simulink library "sm_cable_robot_lib"  (R2021b)
settings: Solver=VariableStepAuto  StartTime=0.0  StopTime=10.0  RelTol=1e-3
undefined symbols (not defined in the file or in its folder): Hand, Left, Right, X, Y, Z
libraries: sm_lib x71, $bdroot x22
(part 1 of 3)
Description:
  | Cable Robot Library
settings Model: Creator=The MathWorks, Inc.  LastModifiedBy=The MathWorks, Inc.
settings SolverCC: AlgebraicLoopSolver=TrustRegion  DecoupledContinuousIntegration=on  MinimalZcImpactIntegration=on
settings DataIOCC: ReturnWorkspaceOutputs=off
settings DebuggingCC: SFMachineParentedDataDiag=warning  ArithmeticOperatorsInVariantConditions=warning
settings SFSimCC: SimUseLocalCustomCode=off  CustomCodeUndefinedFunction=UseInterfaceOnly
settings RTWCC: RTWUseLocalCustomCode=off

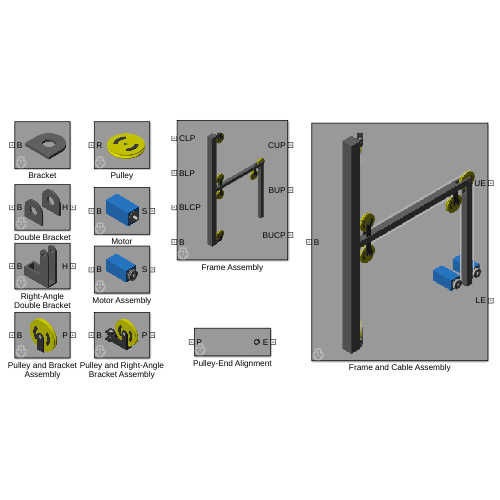
[thumbnail: Simulink's stored preview of the top-level diagram]
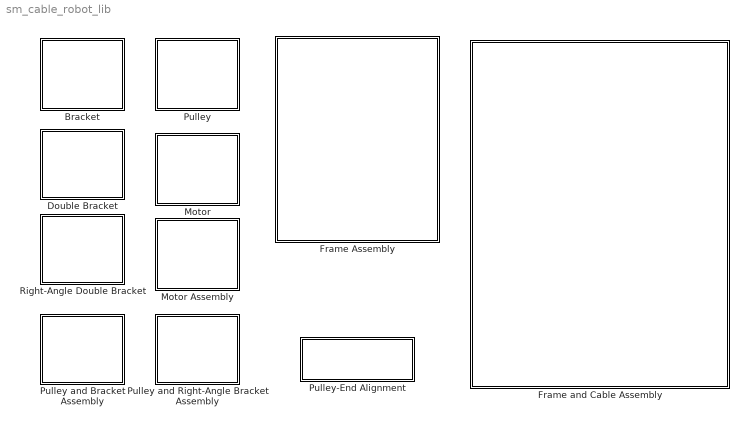
== system sm_cable_robot_lib ==
  Bracket : Subsystem  mask(Bracket){height=0.1, width=0.1, thickness=0.01, holeOffset=0.05, holeRadius=0.02, rho=2700, color=[0.5 0.5 0.5]}
      mask prompts: height "Height (m)"; width "Width (m)"; thickness "Thickness (m)"; holeOffset "Hole Offset (m)"; holeRadius "Hole Radius (m)"; rho "Density (kg/m^3)"; color "Color [r g b]"
      mask help:
      | This block models a bracket element.
      |
      | Port B corresponds to the center point of the base face.
      mask init:
      | y = height - 0.5*width;
      | 
      | outerVertices = ...
      |   [          0      0;...
      |      0.5*width      0;...
      |      0.5*width      y;...
      |      0.5*width height;...
      |     -0.5*width height;...
      |     -0.5*width      y;...
      |     -0.5*width      0;...
      |              0      0];
      | 
      | outer = simmechanics.demohelpers.round_corners(...
      |   outerVertices, [4 5], 0.5*width, 10);
      | 
      | holeTheta = linspace(1.5*pi, -0.5*pi, 20);
      | 
      | hole = [holeRadius*cos(holeTheta);...
      |         holeRadius*sin(holeTheta)+holeOffset]';
      | 
      | crossSection = [hole; outer];
      mask DialogControl Tab1 Prompt: Dimensions
      mask DialogControl Tab2 Prompt: Material Properties
      mask Display: image(fullfile(matlabroot,'toolbox','physmod','sm','smdemos','cable_robot','images','sm_cable_robot_bracket.png'));
  Double Bracket : Subsystem  mask(Double Bracket){height=0.1, width=0.1, thickness=0.01, offset=0.1, holeOffset=0.05, holeRadius=0.02, rho=7800, color=[0.5 0.5 0.5]}
      mask prompts: height "Height (m)"; width "Width (m)"; thickness "Thickness (m)"; offset "Offset (m)"; holeOffset "Hole Offset (m)"; holeRadius "Hole Radius (m)"; rho "Density (kg/m^3)"; color "Color [r g b]"
      mask help:
      | This block models a double bracket element.
      |
      | Port B corresponds to the midpoint between the base faces of the two elements. Port H corresponds to the midpoint between the two holes.
      mask DialogControl Tab1 Prompt: Dimensions
      mask DialogControl Tab2 Prompt: Material Properties
      mask Display: image(fullfile(matlabroot,'toolbox','physmod','sm','smdemos','cable_robot','images','sm_cable_robot_double_bracket.png'));
  Frame Assembly : Subsystem  mask(Frame Assembly){frameType=Right-Hand, frameColumnWidth=0.05, frameColumnHeight=1, frameBeamWidth=0.03, frameBeamLength=0.625, bracketWidth=0.02, bracketThickness=0.005, bracketTolerance=0.002, swivelHoleRadius=0.005, rightAngleBracketWidth=0.015, pulleyRadius=0.04, pulleyThickness=0.01, pulleyHoleRadius=0.005, pulleyGrooveDepth=0.005, pulleyGrooveWidth=0.005, pulleyGrooveAngle=25, pulleyFrameGap=0.02, frameRho=7800, pulleyRho=7800, pinRho=7800, frameColor=[0.5 0.5 0.5], bracketColor=[0.3 0.3 0.3], pulleyColor=[1.0 1.0 0.0], pulleyMarkerColor=[0.3 0.3 0.3], pinColor=[0.9 0.9 0.9]}
      mask prompts: frameType "Type"; frameColumnWidth "Column Width (m)"; frameColumnHeight "Column Height (m)"; frameBeamWidth "Beam Width (m)"; frameBeamLength "Beam Length (m)"; bracketWidth "Width (m)"; bracketThickness "Thickness (m)"; bracketTolerance "Tolerance (m)"; swivelHoleRadius "Swivel Hole Radius (m)"; rightAngleBracketWidth "Right-Bracket Width (m)"; pulleyRadius "Radius (m)"; pulleyThickness "Thickness (m)"; pulleyHoleRadius "Hole Radius (m)"; pulleyGrooveDepth "Groove Depth (m)"; pulleyGrooveWidth "Groove Width (m)"; pulleyGrooveAngle "Groove Angle (m)"; pulleyFrameGap "Frame Gap (m)"; frameRho "Frame Density (kg/m^3)"; pulleyRho "Pulley Density (kg/m^3)"; pinRho "Pin Density (kg/m^3)"; frameColor "Frame Color [r g b]"; bracketColor "Bracket Color [r g b]"; pulleyColor "Pulley Color [r g b]"; pulleyMarkerColor "Pulley Marker Color [r g b]"; pinColor "Pin Color [r g b]"
      mask help:
      | This block models the complete frame assembly of the cable robot. It includes all the pulleys and their joints that provide the degrees of freedom.
      |
      | Port B corresponds to the base corner of the frame column. The remaining ports correspond to the pulley reference frames.
      mask init:
      | % Frame Type
      | if frameType == 1
      |   dir = +1;
      | else
      |   dir = -1;
      | end
      | 
      | % Pulley
      | pulleyPitchRadius = pulleyRadius - 0.5 * pulleyGrooveDepth;
      | 
      | % Swivel Bracket
      | swivelBracketHoleOffset = bracketWidth - 1.5 * swivelHoleRadius;
      | swivelBracketOffset     = rightAngleBracketWidth + bracketThickness;
      | swivelBracketWidth      = pulleyThickness + 2 * bracketTolerance + 2 * bracketThickness;
      | 
      | % Right-Angle Bracket
      | rightAngleBracketHoleOffset = pulleyRadius + bracketThickness + bracketTolerance;
      | rightAngleBracketHeight     = rightAngleBracketHoleOffset + 1.5 * pulleyHoleRadius;
      | rightAngleBracketLegLength  = pulleyPitchRadius +0.5 * bracketThickness - 0.5 * rightAngleBracketWidth - swivelBracketHoleOffset;
      | 
      | % Beam Pulleys and Brackets
      | beamLeftPulleyOffset  = pulleyPitchRadius + swivelBracketHoleOffset;
      | beamBracketHoleOffset = pulleyRadius + pulleyFrameGap;
      | beamBracketHeight     = beamBracketHoleOffset + 1.5 * pulleyHoleRadius;
      | beamBracketOffset     = pulleyThickness + 2 * bracketTolerance + bracketThickness;
      | 
      | % Column
      | columnDimension = [frameColumnWidth frameColumnWidth frameColumnHeight];
      | columnBaseOffset = dir * 0.5 * frameColumnWidth;
      | 
      | columnLowerPulleyOffset = ...
      |   [dir * 0.5 * (frameColumnWidth - frameBeamWidth), ...
      |    0, ...
      |    bracketTolerance + 0.5 * (bracketThickness + swivelBracketOffset)];
      | 
      | columnUpperPulleyOffset    = columnLowerPulleyOffset;
      | columnUpperPulleyOffset(3) = -columnUpperPulleyOffset(3);
      | 
      | % Beam and Strut
      | beamOffset = dir * 0.5 * (frameColumnWidth - frameBeamWidth);
      | 
      | notchLength = 1.1 * pulleyRadius + frameBeamWidth;
      | framePlateThickness = 0.5 * (frameBeamWidth - pulleyThickness - 2 * bracketTolerance);
      | 
      | beamDimension      = [frameBeamWidth, frameBeamWidth, frameBeamLength - notchLength];
      | beamPlateDimension = [framePlateThickness, frameBeamWidth, notchLength - frameBeamWidth];
      | strutDimension     = [frameBeamWidth, frameBeamWidth, 0.5 * (frameColumnHeight + frameBeamWidth) - notchLength];
      | 
      | holePoints = linspace(pi, -pi, 20);
      | strutPlateHole = [pulleyHoleRadius * cos(holePoints) + 0.5 * frameBeamWidth;...
      |                   pulleyHoleRadius * sin(holePoints)]';
      | 
      | strutPlateCrossSection = [            ...
      |   0          , 0;                     ...
      |   strutPlateHole;                     ...
      |   0          , 0;                     ...
      |   0          , -0.5 * frameBeamWidth; ...
      |   notchLength, -0.5 * frameBeamWidth; ...
      |   notchLength, +0.5 * frameBeamWidth; ...
      |   0          , +0.5 * frameBeamWidth];
      | 
      | % Beam Corner Pulleys
      | beamLowerCornerPulleyOffset = pulleyPitchRadius + pulleyFrameGap - beamPlateDimension(3);
      | beamUpperCornerPulleyOffset = [-(beamPlateDimension(3) + 0.5 * frameBeamWidth), 0, -0.5 * frameBeamWidth];
      mask TypeOptions frameType: Right-Hand | Left-Hand
      mask DialogControl Tab1 Prompt: Frame Dimensions
      mask DialogControl Tab2 Prompt: Bracket Dimensions
      mask DialogControl Tab3 Prompt: Pulley Dimensions
      mask DialogControl Tab4 Prompt: Material Properties
      mask Display: image(fullfile(matlabroot,'toolbox','physmod','sm','smdemos','cable_robot','images','sm_cable_robot_frame_assembly.png'));
  Frame and Cable Assembly : Subsystem  mask(Frame and Cable Assembly){frameType=Right-Hand, frameColumnWidth=0.05, frameColumnHeight=1, frameBeamWidth=0.03, frameBeamLength=0.625, bracketWidth=0.02, bracketThickness=0.005, bracketTolerance=0.002, swivelHoleRadius=0.005, rightBracketWidth=0.015, motorWidth=0.05, motorHeight=0.05, motorDepth=0.1, motorShaftRadius=0.005, motorShaftLength=0.02, pulleyRadius=0.04, pulleyThickness=0.01, pulleyHoleRadius=0.005, pulleyGrooveDepth=0.004, pulleyGrooveWidth=0.005, pulleyGrooveAngle=25, pulleyFrameGap=0.02, spoolRadius=0.02, spoolThickness=0.01, spoolGrooveDepth=0.004, spoolGrooveWidth=0.005, spoolGrooveAngle=25, ringMajorRadius=0.003, ringMinorRadius=0.001, frameRho=7800, pinRho=7800, motorHousingRho=7800, motorShaftRho=7800, pulleyRho=7800, spoolRho=7800, ringRho=7800, frameColor=[0.5 0.5 0.5], bracketColor=[0.3 0.3 0.3], pinColor=[0.9 0.9 0.9], motorHousingColor=[0.2 0.6 1.0], motorFlangeColor=[0.7 0.7 0.7], motorShaftColor=[0.9 0.9 0.9], pulleyColor=[1.0 1.0 0.0], pulleyMarkerColor=[0.3 0.3 0.3], spoolColor=[0.7 0.7 0.7], spoolMarkerColor=[0.3 0.3 0.3], cableColor=[0.7 0.7 0.7], ringColor=[0.3 0.3 0.3]}
      mask prompts: frameType "Frame Type"; frameColumnWidth "Column Width (m)"; frameColumnHeight "Column Height (m)"; frameBeamWidth "Beam Width (m)"; frameBeamLength "Beam Length (m)"; bracketWidth "Width (m)"; bracketThickness "Thickness (m)"; bracketTolerance "Tolerance (m)"; swivelHoleRadius "Swivel Hole Radius (m)"; rightBracketWidth "Right-Bracket Width (m)"; motorWidth "Width (m)"; motorHeight "Height (m)"; motorDepth "Depth (m)"; motorShaftRadius "Shaft Radius (m)"; motorShaftLength "Shaft Length (m)"; pulleyRadius "Radius (m)"; pulleyThickness "Thickness (m)"; pulleyHoleRadius "Hole Radius (m)"; pulleyGrooveDepth "Groove Depth (m)"; pulleyGrooveWidth "Groove Width (m)"; pulleyGrooveAngle "Groove Angle (deg)"; pulleyFrameGap "Frame Gap (m)"; spoolRadius "Radius (m)"; spoolThickness "Thickness (m)"; spoolGrooveDepth "Groove Depth (m)"; spoolGrooveWidth "Groove Width (m)"; spoolGrooveAngle "Groove Angle (deg)"; ringMajorRadius "Major Radius (m)"; ringMinorRadius "Minor Radius (m)"; frameRho "Frame Density (kg/m^3)"; pinRho "Pin Density (kg/m^3)"; motorHousingRho "Motor Housing Density (kg/m^3)"; motorShaftRho "Motor Shaft Density (kg/m^3)"; pulleyRho "Pulley Density (kg/m^3)"; spoolRho "Spool Density (kg/m^3)"; ringRho "Connector Ring Density (kg/m^3)"; frameColor "Frame Color [r g b]"; bracketColor "Bracket Color [r g b]"; pinColor "Pin Color [r g b]"; motorHousingColor "Motor Housing Color [r g b]"; motorFlangeColor "Motor Flange Color [r g b]"; motorShaftColor "Motor Shaft Color [r g b]"; pulleyColor "Pulley Color [r g b]"; pulleyMarkerColor "Pulley Marker Color [r g b]"; spoolColor "Spool Color [r g b]"; spoolMarkerColor "Spool Marker Color [r g b]"; cableColor "Cable Color [r g b]"; ringColor "Connector Ring Color [r g b]"
      mask help:
      | This block models the complete frame and belt-cable circuits of the cable robot. It includes all the pulleys, their joints, the upper and lower motor assemblies, and the upper and lower belt-cable circuits.
      |
      | Port B corresponds to the base corner of the frame column. Ports UE and LE correspond to the belt-cable ends of the upper and lower belt-cable circuits, respectively.
      mask init:
      | blk = gcb;
      | 
      | % Initialize variables to prevent errors from SET_PARAM calls below
      | lowerMotorOffset = [];
      | upperMotorOffset = [];
      | 
      | if frameType == 1
      |   dir = +1;
      |   set_param([blk '/Frame Assembly'],'frameType','Right-Hand');
      |   set_param([blk '/Lower Cable Circuit/Lower Motor Assembly'],'spoolAlignment','Left-Hand');
      |   set_param([blk '/Lower Cable Circuit/Lower Motor xForm'],'BaseAlignAxisA','+X');
      |   set_param([blk '/Upper Cable Circuit/Upper Motor Assembly'],'spoolAlignment','Right-Hand');
      |   set_param([blk '/Upper Cable Circuit/Upper Motor xForm'],'BaseAlignAxisA','+X');
      | else
      |   dir = -1;
      |   set_param([blk '/Frame Assembly'],'frameType','Left-Hand');
      |   set_param([blk '/Lower Cable Circuit/Lower Motor Assembly'],'spoolAlignment','Right-Hand');
      |   set_param([blk '/Lower Cable Circuit/Lower Motor xForm'],'BaseAlignAxisA','-X');
      |   set_param([blk '/Upper Cable Circuit/Upper Motor Assembly'],'spoolAlignment','Left-Hand');
      |   set_param([blk '/Upper Cable Circuit/Upper Motor xForm'],'BaseAlignAxisA','-X');
      | end
      | 
      | pulleyPitchRadius = pulleyRadius - 0.5 * pulleyGrooveDepth;
      | spoolPitchRadius  = spoolRadius  - 0.5 * spoolGrooveDepth;
      | 
      | lowerMotorOffset = ...
      |   [-dir * 0.5 * (motorDepth + motorShaftLength + frameBeamWidth),...
      |    frameColumnWidth + frameBeamLength - frameBeamWidth - spoolPitchRadius - pulleyFrameGap,...
      |    0];
      | 
      | upperMotorOffset = ...
      |   [lowerMotorOffset(1),...
      |    frameColumnWidth + frameBeamLength + pulleyPitchRadius + spoolPitchRadius - 0.5 * frameBeamWidth,...
      |    0];
      mask TypeOptions frameType: Right-Hand | Left-Hand
      mask DialogControl Tab1 Prompt: Frame Dimensions
      mask DialogControl Tab2 Prompt: Bracket Dimensions
      mask DialogControl Tab3 Prompt: Motor Dimensions
      mask DialogControl Tab4 Prompt: Pulley Dimensions
      mask DialogControl Tab5 Prompt: Spool Dimensions
      mask DialogControl Tab6 Prompt: Connector Ring Dimensions
      mask DialogControl Tab7 Prompt: Material Properties
      mask Display: image(fullfile(matlabroot,'toolbox','physmod','sm','smdemos','cable_robot','images','sm_cable_robot_frame_cable_assembly.png'));
  Motor : Subsystem  mask(Motor){width=0.05, height=0.05, depth=0.1, shaftRadius=0.005, shaftLength=0.02, housingRho=7800, shaftRho=7800, housingColor=[0.2 0.6 1.0], flangeColor=[0.7 0.7 0.7], shaftColor=[0.9 0.9 0.9]}
      mask prompts: width "Width (m)"; height "Height (m)"; depth "Depth (m)"; shaftRadius "Shaft Radius (m)"; shaftLength "Shaft Length (m)"; housingRho "Housing Density (kg/m^3)"; shaftRho "Shaft Density (kg/m^3)"; housingColor "Housing Color [r g b]"; flangeColor "Flange Color [r g b]"; shaftColor "Shaft Color [r g b]"
      mask help:
      | This block models a motor. It includes the motor shaft which is connected to the motor housing through a revolute joint.
      |
      | Port B corresponds to the centerpoint of bottom face of the housing. Port S corresponds to the centerpoint of the motor shaft.
      mask init:
      | if (width < height)
      |   flangeRadius = 0.4 * width;
      | else
      |   flangeRadius = 0.4 * height;
      | end
      | 
      | flangeThickness = 1e-3;
      mask DialogControl Tab1 Prompt: Dimensions
      mask DialogControl Tab2 Prompt: Material Properties
      mask Display: image(fullfile(matlabroot,'toolbox','physmod','sm','smdemos','cable_robot','images','sm_cable_robot_motor.png'));
  Motor Assembly : Subsystem  mask(Motor Assembly){motorWidth=0.05, motorHeight=0.05, motorDepth=0.1, motorShaftRadius=0.005, motorShaftLength=0.02, spoolAlignment=Right-Hand, spoolRadius=0.02, spoolThickness=0.01, spoolGrooveDepth=0.004, spoolGrooveWidth=0.005, spoolGrooveAngle=25, motorHousingRho=7800, motorShaftRho=7800, spoolRho=7800, motorHousingColor=[0.2 0.6 1.0], motorFlangeColor=[0.7 0.7 0.7], motorShaftColor=[0.9 0.9 0.9], spoolColor=[0.7 0.7 0.7], spoolMarkerColor=[0.3 0.3 0.3]}
      mask prompts: motorWidth "Width (m)"; motorHeight "Height (m)"; motorDepth "Depth (m)"; motorShaftRadius "Shaft Radius (m)"; motorShaftLength "Shaft Length (m)"; spoolAlignment "Spool Alignment"; spoolRadius "Radius (m)"; spoolThickness "Thickness (m)"; spoolGrooveDepth "Groove Depth (m)"; spoolGrooveWidth "Groove Width (m)"; spoolGrooveAngle "Groove Angle (deg)"; motorHousingRho "Motor Housing Density (kg/m^3)"; motorShaftRho "Motor Shaft Density (kg/m^3)"; spoolRho "Spool Density (kg/m^3)"; motorHousingColor "Motor Housing Color [r g b]"; motorFlangeColor "Motor Flange Color [r g b]"; motorShaftColor "Motor Shaft Color [r g b]"; spoolColor "Spool Color [r g b]"; spoolMarkerColor "Spool Marker Color [r g b]"
      mask help:
      | This block models a motor and spool assembly. The spool is rigidly connected to the motor shaft.
      |
      | Port B corresponds to the centerpoint of the bottom face of the housing. Port S corresponds to the reference frame of the spool.
      mask init:
      | blk = gcb;
      | 
      | if spoolAlignment == 1
      |   set_param([blk '/Spool Alignment'],'BaseAlignAxisA','+Z');
      | else
      |   set_param([blk '/Spool Alignment'],'BaseAlignAxisA','-Z');
      | end
      mask TypeOptions spoolAlignment: Right-Hand | Left-Hand
      mask DialogControl Tab1 Prompt: Motor Dimensions
      mask DialogControl Tab2 Prompt: Spool Dimensions
      mask DialogControl Tab3 Prompt: Material Properties
      mask Display: image(fullfile(matlabroot,'toolbox','physmod','sm','smdemos','cable_robot','images','sm_cable_robot_motor_assembly.png'));
  Pulley : Subsystem  mask(Pulley){radius=0.04, thickness=0.01, holeRadius=0.005, grooveDepth=0.004, grooveWidth=0.005, grooveAngle=25, rho=7800, color=[1.0 1.0 0.0], markerColor=[0.3 0.3 0.3]}
      mask prompts: radius "Radius (m)"; thickness "Thickness (m)"; holeRadius "Hole Radius (m)"; grooveDepth "Groove Depth (m)"; grooveWidth "Groove Width (m)"; grooveAngle "Groove Angle (deg)"; rho "Density (kg/m^3)"; color "Color [r g b]"; markerColor "Marker Color [r g b]"
      mask help:
      | This block models a pulley solid body.
      |
      | Port R corresponds with the centerpoint of the pulley hole.
      mask init:
      | crossSection = [...
      |   radius              ,  0.5 * thickness;...
      |   holeRadius          ,  0.5 * thickness;...
      |   holeRadius          , -0.5 * thickness;...
      |   radius              , -0.5 * thickness;...
      |   radius              , -0.5 * grooveWidth;...
      |   radius - grooveDepth, -0.5 * grooveWidth + grooveDepth * tand(grooveAngle);...
      |   radius - grooveDepth,  0.5 * grooveWidth - grooveDepth * tand(grooveAngle);...
      |   radius              ,  0.5 * grooveWidth];
      | 
      | markerWidth     = 0.25 * (radius - holeRadius);
      | markerOffset    = holeRadius + 0.5 * (radius - holeRadius);
      | markerThickness = 1e-3;
      | markerRevAngle  = 90;
      | 
      | markerCrossSection = [...
      |   markerOffset - 0.5 * markerWidth, 0;...
      |   markerOffset + 0.5 * markerWidth, 0;...
      |   markerOffset + 0.5 * markerWidth, markerThickness;...
      |   markerOffset - 0.5 * markerWidth, markerThickness];
      mask DialogControl Tab1 Prompt: Dimensions
      mask DialogControl Tab2 Prompt: Material Properties
      mask Display: image(fullfile(matlabroot,'toolbox','physmod','sm','smdemos','cable_robot','images','sm_cable_robot_pulley.png'));
  Pulley and Bracket Assembly : Subsystem  mask(Pulley and Bracket Assembly){bracketHeight=0.05, bracketWidth=0.02, bracketThickness=0.002, bracketOffset=0.02, bracketHoleOffset=0.04, pulleyRadius=0.04, pulleyThickness=0.01, pulleyHoleRadius=0.005, pulleyGrooveDepth=0.004, pulleyGrooveWidth=0.005, pulleyGrooveAngle=25, bracketRho=7800, pulleyRho=7800, pinRho=7800, bracketColor=[0.3 0.3 0.3], pulleyColor=[1.0 1.0 0.0], pulleyMarkerColor=[0.3 0.3 0.3], pinColor=[0.9 0.9 0.9]}
      mask prompts: bracketHeight "Height (m)"; bracketWidth "Width (m)"; bracketThickness "Thickness (m)"; bracketOffset "Offset (m)"; bracketHoleOffset "Hole Offset (m)"; pulleyRadius "Radius (m)"; pulleyThickness "Thickness (m)"; pulleyHoleRadius "Hole Radius (m)"; pulleyGrooveDepth "Groove Depth (m)"; pulleyGrooveWidth "Groove Width (m)"; pulleyGrooveAngle "Groove Angle (deg)"; bracketRho "Bracket Density (kg/m^3)"; pulleyRho "Pulley Density (kg/m^3)"; pinRho "Pin Density (kg/m^3)"; bracketColor "Bracket Color [r g b]"; pulleyColor "Pulley Color [r g b]"; pulleyMarkerColor "Pulley Marker Color [r g b]"; pinColor "Pin Color [r g b]"
      mask help:
      | This block models a pulley and bracket assembly. The pulley is connected to the bracket via a revolute joint. The pulley axis is aligned with the bracket hole axis.
      |
      | Port B corresponds to the base of the bracket. Port P corresponds to the reference frame of the pulley.
      mask init:
      | pinLength = bracketOffset + bracketThickness;
      mask DialogControl Tab1 Prompt: Bracket Dimensions
      mask DialogControl Tab2 Prompt: Pulley Dimensions
      mask DialogControl Tab3 Prompt: Material Properties
      mask Display: image(fullfile(matlabroot,'toolbox','physmod','sm','smdemos','cable_robot','images','sm_cable_robot_pulley_bracket_assembly.png'));
  Pulley and Right-Angle Bracket Assembly : Subsystem  mask(Pulley and Right-Angle Bracket Assembly){baseBracketHeight=0.022, baseBracketWidth=0.022, baseBracketThickness=0.005, baseBracketOffset=0.024, baseBracketHoleOffset=0.012, baseBracketHoleRadius=0.005, rightBracketWidth=0.015, rightBracketHeight=0.06, rightBracketLegLength=0.04, rightBracketHoleOffset=0.05, pulleyRadius=0.04, pulleyThickness=0.01, pulleyHoleRadius=0.005, pulleyGrooveDepth=0.004, pulleyGrooveWidth=0.005, pulleyGrooveAngle=25, bracketRho=7800, pulleyRho=7800, pinRho=7800, bracketColor=[0.3 0.3 0.3], pulleyColor=[1.0 1.0 0.0], pulleyMarkerColor=[0.3 0.3 0.3], pinColor=[0.9 0.9 0.9]}
      mask prompts: baseBracketHeight "Height (m)"; baseBracketWidth "Width (m)"; baseBracketThickness "Thickness (m)"; baseBracketOffset "Offset (m)"; baseBracketHoleOffset "Hole Offset (m)"; baseBracketHoleRadius "Hole Radius (m)"; rightBracketWidth "Width (m)"; rightBracketHeight "Height (m)"; rightBracketLegLength "Leg Length (m)"; rightBracketHoleOffset "Hole Offset (m)"; pulleyRadius "Radius (m)"; pulleyThickness "Thickness (m)"; pulleyHoleRadius "Hole Radius (m)"; pulleyGrooveDepth "Groove Depth (m)"; pulleyGrooveWidth "Groove Width (m)"; pulleyGrooveAngle "Groove Angle (deg)"; bracketRho "Bracket Density (kg/m^3)"; pulleyRho "Pulley Density (kg/m^3)"; pinRho "Pin Density (kg/m^3)"; bracketColor "Bracket Color [r g b]"; pulleyColor "Pulley Color [r g b]"; pulleyMarkerColor "Pulley Marker Color [r g b]"; pinColor "Pin Color [r g b]"
      mask help:
      | This blocks models a pulley and right-angle bracket assembly. The pulley is connected to the right-angle bracket via a revolute joint. The pulley axis is aligned with the right-angle bracket hole axis. The right-angle bracket is connected to a pair of double brackets, with the right-angle bracket rigidly connected to one, and the other is connected to the first double bracket via a revolute joint.
      |
      | Port B corresponds to the base of the second double bracket. Port P corresponds to the reference frame of the pulley.
      mask init:
      | rightBracketOffset    = baseBracketWidth - baseBracketThickness;
      | follBracketOffset     = baseBracketOffset - 2 * baseBracketThickness;
      | follBracketHeight     = baseBracketHeight - baseBracketThickness;
      | follBracketHoleOffset = baseBracketHoleOffset - baseBracketThickness;
      | 
      | swivelPinLength       = baseBracketOffset  + baseBracketThickness;
      | pulleyPinLength       = rightBracketOffset + baseBracketThickness;
      mask DialogControl Tab1 Prompt: Base Bracket Dimensions
      mask DialogControl Tab2 Prompt: Right-Angle Bracket Dimensions
      mask DialogControl Tab3 Prompt: Pulley Dimensions
      mask DialogControl Tab4 Prompt: Material Properties
      mask Display: image(fullfile(matlabroot,'toolbox','physmod','sm','smdemos','cable_robot','images','sm_cable_robot_pulley_right_bracket_assembly.png'));
  Pulley-End Alignment : Subsystem  mask(Pulley-End Alignment){majorRadius=0.003, minorRadius=0.001, rho=7800, color=[0.3 0.3 0.3]}
      mask prompts: majorRadius "Ring Major Radius (m)"; minorRadius "Ring Minor Radius (m)"; rho "Ring Density (kg/m^3)"; color "Ring Color [r g b]"
      mask help:
      | This block models the enforced alignment between the belt-cable end attached to the mover and the corresponding column pulley. The block maintains the alignment between the belt-cable and the column pulley such that the belt-cable is always in the x-y plane of the column pulley.
      |
      | Port P corresponds to the pulley reference frame. Port E corresponds to the belt-cable end reference frame.
      mask init:
      | theta = linspace(0, 2 * pi, 20);
      | 
      | crossSection = [minorRadius * cos(theta) + majorRadius;...
      |                 minorRadius * sin(theta)]';
      mask DialogControl Tab1 Prompt: Dimensions
      mask DialogControl Tab2 Prompt: Material Properties
      mask Display: image(fullfile(matlabroot,'toolbox','physmod','sm','smdemos','cable_robot','images','sm_cable_robot_pulley_end_alignment.png'));
  Right-Angle Double Bracket : Subsystem  mask(Right-Angle Double Bracket){height=1, width=0.25, thickness=0.05, legLength=0.5, offset=0.25, holeOffset=0.85, holeRadius=0.05, rho=7800, color=[0.5 0.5 0.5]}
      mask prompts: height "Height (m)"; width "Width (m)"; thickness "Thickness (m)"; legLength "Leg Length (m)"; offset "Offset (m)"; holeOffset "Hole Offset (m)"; holeRadius "Hole Radius (m)"; rho "Density (kg/m^3)"; color "Color [r g b]"
      mask help:
      | This block models a right-angle double bracket.
      |
      | Port B corresponds to the centerpoint of the left-end base face. Port H corresponds to the midpoint between the two holes.
      mask init:
      | legDimension   = [legLength width thickness];
      | frontLegOffset = ...
      |   [-0.5 * width - 0.5 * legLength, -0.5 * offset, 0.5 * width];
      | 
      | rearLegOffset    = frontLegOffset;
      | rearLegOffset(2) = -rearLegOffset(2);
      | 
      | basePlateDimension = [0.5 * thickness, offset + thickness, width];
      | basePlateOffset    = ...
      |   [-0.5 * width - legLength - 0.25 * thickness, 0, 0.5 * width];
      | 
      | bottomDimension = ...
      |   [width + legLength, offset - thickness, thickness];
      | bottomOffset    = ...
      |   [0.5 * width - 0.5 * bottomDimension(1), 0, 0.5 * thickness];
      mask DialogControl Tab1 Prompt: Dimensions
      mask DialogControl Tab2 Prompt: Material Properties
      mask Display: image(fullfile(matlabroot,'toolbox','physmod','sm','smdemos','cable_robot','images','sm_cable_robot_right_angle_bracket.png'));

== system sm_cable_robot_lib/Bracket ==
  Bracket : sm_lib/Body Elements/Extruded Solid  GraphicAmbientColor=[0.15 0.15 0.15 1.0]  BasedOnType=Density  CenterOfMass=[0 0 0]  CenterOfMassUnits=m  GraphicDiffuseColor=color  ExportConvexHullGeometry=off  ExtrusionCrossSection=crossSection  ExtrusionCrossSectionUnits=m  Density=rho  DensityUnits=kg/m^3  DoExposeReferenceFrame=on  GraphicEmissiveColor=[0.0 0.0 0.0 1.0]  ExportEntireGeometry=off  ExtrusionLength=thickness  ExtrusionLengthUnits=m  ExtrusionType=General  SerializedFrames=<Frames/>  MarkerShape=Sphere  MarkerSize=10  GraphicType=FromGeometry  InertiaType=CalculateFromGeometry  Mass=1  MassUnits=kg  MomentsOfInertia=[1 1 1]  MomentsOfInertiaUnits=kg*m^2  PolygonNumSides=3  GraphicOpacity=1.0  PolygonOuterRadius=1  PolygonOuterRadiusUnits=m  ProductsOfInertia=[1 1 1]  ProductsOfInertiaUnits=kg*m^2  GraphicShininess=75  GraphicSpecularColor=[0.5 0.5 0.5 1.0]  GraphicVisPropType=SimpleVisualProperties
  B : PMIOPort  Side=Left
  connections:
  Bracket/RConn1 -- B/RConn1

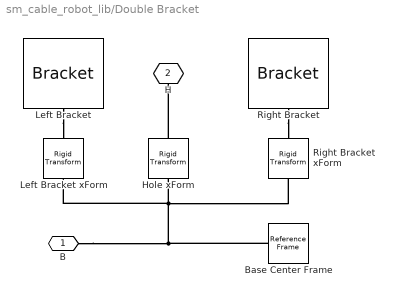
== system sm_cable_robot_lib/Double Bracket ==
  Base Center Frame : sm_lib/Frames and Transforms/Reference Frame
  Hole xForm : sm_lib/Frames and Transforms/Rigid Transform  TranslationMethod=StandardAxis  TranslationStandardOffset=holeOffset  TranslationLengthUnit=m  TranslationStandardAxis=+Z  TranslationCartesianOffset=[0 0 0]  TranslationROffset=0  TranslationROffsetUnits=m  TranslationZOffset=0  TranslationZOffsetUnits=m  TranslationThetaOffset=0  TranslationThetaOffsetUnits=deg  RotationMethod=AlignedAxes  RotationAngleUnits=deg  RotationStandardAxis=+X  RotationAngle=90  RotationArbitraryAxis=[0 0 1]  FollAlignAxisA=+X  BaseAlignAxisA=+X  FollAlignAxisB=+Y  BaseAlignAxisB=+Z  RotationSequenceAxes=FollowerAxes  RotationSequence=XYX  RotationSequenceAngles=[0 0 0]  RotationSequenceAnglesUnits=deg  RotationMatrix=[1 0 0; 0 1 0; 0 0 1]
  Left Bracket : $bdroot/Bracket  height=height  width=width  thickness=thickness  holeOffset=holeOffset  holeRadius=holeRadius  rho=rho  color=color
  Left Bracket xForm : sm_lib/Frames and Transforms/Rigid Transform  TranslationMethod=StandardAxis  TranslationStandardOffset=0.5*offset  TranslationLengthUnit=m  TranslationStandardAxis=-Y  TranslationCartesianOffset=[0 0 0]  TranslationROffset=0  TranslationROffsetUnits=m  TranslationZOffset=0  TranslationZOffsetUnits=m  TranslationThetaOffset=0  TranslationThetaOffsetUnits=deg  RotationMethod=AlignedAxes  RotationAngleUnits=deg  RotationStandardAxis=+X  RotationAngle=90  RotationArbitraryAxis=[0 0 1]  FollAlignAxisA=+X  BaseAlignAxisA=+X  FollAlignAxisB=+Y  BaseAlignAxisB=+Z  RotationSequenceAxes=FollowerAxes  RotationSequence=XYX  RotationSequenceAngles=[0 0 0]  RotationSequenceAnglesUnits=deg  RotationMatrix=[1 0 0; 0 1 0; 0 0 1]
  Right Bracket : $bdroot/Bracket  height=height  width=width  thickness=thickness  holeOffset=holeOffset  holeRadius=holeRadius  rho=rho  color=color
  Right Bracket xForm : sm_lib/Frames and Transforms/Rigid Transform  TranslationMethod=StandardAxis  TranslationStandardOffset=0.5*offset  TranslationLengthUnit=m  TranslationStandardAxis=+Y  TranslationCartesianOffset=[0 0 0]  TranslationROffset=0  TranslationROffsetUnits=m  TranslationZOffset=0  TranslationZOffsetUnits=m  TranslationThetaOffset=0  TranslationThetaOffsetUnits=deg  RotationMethod=AlignedAxes  RotationAngleUnits=deg  RotationStandardAxis=+X  RotationAngle=90  RotationArbitraryAxis=[0 0 1]  FollAlignAxisA=+X  BaseAlignAxisA=+X  FollAlignAxisB=+Y  BaseAlignAxisB=+Z  RotationSequenceAxes=FollowerAxes  RotationSequence=XYX  RotationSequenceAngles=[0 0 0]  RotationSequenceAnglesUnits=deg  RotationMatrix=[1 0 0; 0 1 0; 0 0 1]
  B : PMIOPort  Side=Left
  H : PMIOPort  Port=2  Side=Right
  connections:
  Left Bracket/LConn1 -- Left Bracket xForm/RConn1
  Hole xForm/RConn1 -- H/RConn1
  Right Bracket/LConn1 -- Right Bracket xForm/RConn1
  Left Bracket xForm/LConn1 -- Right Bracket xForm/LConn1 -- Base Center Frame/RConn1 -- B/RConn1 -- Hole xForm/LConn1

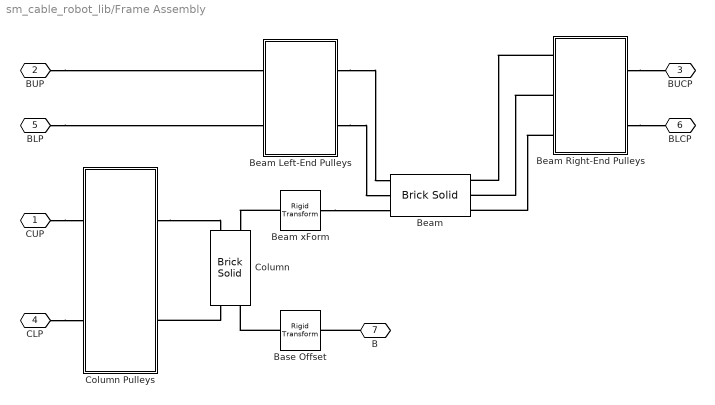
== system sm_cable_robot_lib/Frame Assembly ==
  Base Offset : sm_lib/Frames and Transforms/Rigid Transform  TranslationMethod=StandardAxis  TranslationStandardOffset=columnBaseOffset  TranslationLengthUnit=m  TranslationStandardAxis=+X  TranslationCartesianOffset=[0 0 0]  TranslationROffset=0  TranslationROffsetUnits=m  TranslationZOffset=0  TranslationZOffsetUnits=m  TranslationThetaOffset=0  TranslationThetaOffsetUnits=deg  RotationMethod=None  RotationAngleUnits=deg  RotationStandardAxis=+Z  RotationAngle=0.0  RotationArbitraryAxis=[0 0 1]  FollAlignAxisA=+X  BaseAlignAxisA=+Y  FollAlignAxisB=+Y  BaseAlignAxisB=+Z  RotationSequenceAxes=FollowerAxes  RotationSequence=XYX  RotationSequenceAngles=[0 0 0]  RotationSequenceAnglesUnits=deg  RotationMatrix=[1 0 0; 0 1 0; 0 0 1]
  Beam : sm_lib/Body Elements/Brick Solid  GraphicAmbientColor=[0.15 0.15 0.15 1.0]  BasedOnType=Density  BrickDimensions=beamDimension  BrickDimensionUnits=m  CenterOfMass=[0 0 0]  CenterOfMassUnits=m  GraphicDiffuseColor=frameColor  Density=frameRho  DensityUnits=kg/m^3  DoExposeReferenceFrame=off  GraphicEmissiveColor=[0.0 0.0 0.0 1.0]  ExportEntireGeometry=off  SerializedFrames=<Frames><Frame><Id>Frame1</Id><Value><Name>LU</Name><Origin><Source>GeometricFeature</Source><FeatureName>+y +z curve</FeatureName></Origin><PrimaryAxis><DefinedDirection>+X</DefinedDirection><Source>ReferenceFrame</Source><SourceDirection>-Z</SourceDirection><FeatureName></FeatureName></PrimaryAxis><SecondaryAxis><DefinedDirection>+Z</DefinedDirection><Source>ReferenceFrame</Source><SourceDirection>+Y</SourceDirection><FeatureName></FeatureName></SecondaryAxis></Value></Frame><Frame><Id>Frame2</Id><Value><Name>RR</Name><Origin><Source>GeometricFeature</Source><FeatureName>-z -x curve</FeatureName></Origin><PrimaryAxis><DefinedDirection>+Z</DefinedDirection><Source>ReferenceFrame</Source><SourceDirection>+Z</SourceDirection><FeatureName></FeatureName></PrimaryAxis><SecondaryAxis><DefinedDirection>+X</DefinedDirection><Source>ReferenceFrame</Source><SourceDirection>+X</SourceDirection><FeatureName></FeatureName></SecondaryAxis></Value></Frame><Frame><Id>Frame3</Id><Value><Name>LL</Name><Origin><Source>GeometricFeature</Source><FeatureName>-y +z curve</FeatureName></Origin><PrimaryAxis><DefinedDirection>+Z</DefinedDirection><Source>ReferenceFrame</Source><SourceDirection>-Y</SourceDirection><FeatureName></FeatureName></PrimaryAxis><SecondaryAxis><DefinedDirection>+X</DefinedDirection><Source>ReferenceFrame</Source><SourceDirection>-Z</SourceDirection><FeatureName></FeatureName></SecondaryAxis></Value></Frame><Frame><Id>Frame4</Id><Value><Name>RF</Name><Origin><Source>GeometricFeature</Source><FeatureName>-z +x curve</FeatureName></Origin><PrimaryAxis><DefinedDirection>+Z</DefinedDirection><Source>ReferenceFrame</Source><SourceDirection>+Z</SourceDirection><FeatureName></FeatureName></PrimaryAxis><SecondaryAxis><DefinedDirection>+X</DefinedDirection><Source>ReferenceFrame</Source><SourceDirection>+X</SourceDirection><FeatureName></FeatureName></SecondaryAxis></Value></Frame><Frame><Id>Frame5</Id><Value><Name>L</Name><Origin><Source>GeometricFeature</Source><FeatureName>+z surface</FeatureName></Origin><PrimaryAxis><DefinedDirection>+Z</DefinedDirection><Source>ReferenceFrame</Source><SourceDirection>+Y</SourceDirection><FeatureName></FeatureName></PrimaryAxis><SecondaryAxis><DefinedDirection>+X</DefinedDirection><Source>ReferenceFrame</Source><SourceDirection>+X</SourceDirection><FeatureName></FeatureName></SecondaryAxis></Value></Frame><Frame><Id>Frame6</Id><Value><Name>R</Name><Origin><Source>GeometricFeature</Source><FeatureName>-y -z curve</FeatureName></Origin><PrimaryAxis><DefinedDirection>+Z</DefinedDirection><Source>ReferenceFrame</Source><SourceDirection>-Y</SourceDirection><FeatureName></FeatureName></PrimaryAxis><SecondaryAxis><DefinedDirection>+X</DefinedDirection><Source>ReferenceFrame</Source><SourceDirection>+Z</SourceDirection><FeatureName></FeatureName></SecondaryAxis></Value></Frame></Frames>  MarkerShape=Sphere  MarkerSize=10  GraphicType=FromGeometry  InertiaType=CalculateFromGeometry  Mass=1  MassUnits=kg  MomentsOfInertia=[1 1 1]  MomentsOfInertiaUnits=kg*m^2  GraphicOpacity=1.0  ProductsOfInertia=[0 0 0]  ProductsOfInertiaUnits=kg*m^2  GraphicShininess=75  GraphicSpecularColor=[0.5 0.5 0.5 1.0]  GraphicVisPropType=SimpleVisualProperties
  Beam Left-End Pulleys : Subsystem
      mask Display: image(fullfile(matlabroot,'toolbox','physmod','sm','smdemos','cable_robot','images','sm_cable_robot_frame_beam_left_pulleys.png'));
  Beam Right-End Pulleys : Subsystem
      mask Display:
      | image(fullfile(matlabroot,'toolbox','physmod','sm','smdemos','cable_robot','images','sm_cable_robot_frame_beam_right_pulleys.png'));
      | port_label('lconn',1,'RR');
      | port_label('lconn',2,'RF');
      | port_label('lconn',3,'R');
      | port_label('rconn',1,'BUCP');
      | port_label('rconn',2,'BLCP');
  Beam xForm : sm_lib/Frames and Transforms/Rigid Transform  TranslationMethod=StandardAxis  TranslationStandardOffset=beamOffset  TranslationLengthUnit=m  TranslationStandardAxis=+X  TranslationCartesianOffset=[0 0 0]  TranslationROffset=0  TranslationROffsetUnits=m  TranslationZOffset=0  TranslationZOffsetUnits=m  TranslationThetaOffset=0  TranslationThetaOffsetUnits=deg  RotationMethod=None  RotationAngleUnits=deg  RotationStandardAxis=+Z  RotationAngle=0.0  RotationArbitraryAxis=[0 0 1]  FollAlignAxisA=+X  BaseAlignAxisA=+Y  FollAlignAxisB=+Y  BaseAlignAxisB=+Z  RotationSequenceAxes=FollowerAxes  RotationSequence=XYX  RotationSequenceAngles=[0 0 0]  RotationSequenceAnglesUnits=deg  RotationMatrix=[1 0 0; 0 1 0; 0 0 1]
  Column : sm_lib/Body Elements/Brick Solid  GraphicAmbientColor=[0.15 0.15 0.15 1.0]  BasedOnType=Density  BrickDimensions=columnDimension  BrickDimensionUnits=m  CenterOfMass=[0 0 0]  CenterOfMassUnits=m  GraphicDiffuseColor=frameColor  Density=frameRho  DensityUnits=kg/m^3  DoExposeReferenceFrame=off  GraphicEmissiveColor=[0.0 0.0 0.0 1.0]  ExportEntireGeometry=off  SerializedFrames=<Frames><Frame><Id>Frame1</Id><Value><Name>LP</Name><Origin><Source>GeometricFeature</Source><FeatureName>+y -z curve</FeatureName></Origin><PrimaryAxis><DefinedDirection>+Z</DefinedDirection><Source>ReferenceFrame</Source><SourceDirection>+Z</SourceDirection><FeatureName></FeatureName></PrimaryAxis><SecondaryAxis><DefinedDirection>+X</DefinedDirection><Source>ReferenceFrame</Source><SourceDirection>+X</SourceDirection><FeatureName></FeatureName></SecondaryAxis></Value></Frame><Frame><Id>Frame2</Id><Value><Name>UP</Name><Origin><Source>GeometricFeature</Source><FeatureName>+y +z curve</FeatureName></Origin><PrimaryAxis><DefinedDirection>+Z</DefinedDirection><Source>ReferenceFrame</Source><SourceDirection>+Z</SourceDirection><FeatureName></FeatureName></PrimaryAxis><SecondaryAxis><DefinedDirection>+X</DefinedDirection><Source>ReferenceFrame</Source><SourceDirection>+X</SourceDirection><FeatureName></FeatureName></SecondaryAxis></Value></Frame><Frame><Id>Frame3</Id><Value><Name>B</Name><Origin><Source>GeometricFeature</Source><FeatureName>-y -z curve</FeatureName></Origin><PrimaryAxis><DefinedDirection>+Z</DefinedDirection><Source>ReferenceFrame</Source><SourceDirection>+Z</SourceDirection><FeatureName></FeatureName></PrimaryAxis><SecondaryAxis><DefinedDirection>+X</DefinedDirection><Source>ReferenceFrame</Source><SourceDirection>+X</SourceDirection><FeatureName></FeatureName></SecondaryAxis></Value></Frame><Frame><Id>Frame4</Id><Value><Name>M</Name><Origin><Source>GeometricFeature</Source><FeatureName>+y surface</FeatureName></Origin><PrimaryAxis><DefinedDirection>+Z</DefinedDirection><Source>ReferenceFrame</Source><SourceDirection>+Z</SourceDirection><FeatureName></FeatureName></PrimaryAxis><SecondaryAxis><DefinedDirection>+X</DefinedDirection><Source>ReferenceFrame</Source><SourceDirection>+X</SourceDirection><FeatureName></FeatureName></SecondaryAxis></Value></Frame></Frames>  MarkerShape=Sphere  MarkerSize=10  GraphicType=FromGeometry  InertiaType=CalculateFromGeometry  Mass=1  MassUnits=kg  MomentsOfInertia=[1 1 1]  MomentsOfInertiaUnits=kg*m^2  GraphicOpacity=1.0  ProductsOfInertia=[0 0 0]  ProductsOfInertiaUnits=kg*m^2  GraphicShininess=75  GraphicSpecularColor=[0.5 0.5 0.5 1.0]  GraphicVisPropType=SimpleVisualProperties
  Column Pulleys : Subsystem
      mask Display: image(fullfile(matlabroot,'toolbox','physmod','sm','smdemos','cable_robot','images','sm_cable_robot_frame_column_pulleys.png'));
  CUP : PMIOPort  Side=Right
  BUP : PMIOPort  Port=2  Side=Right
  BUCP : PMIOPort  Port=3  Side=Right
  CLP : PMIOPort  Port=4  Side=Left
  BLP : PMIOPort  Port=5  Side=Left
  BLCP : PMIOPort  Port=6  Side=Left
  B : PMIOPort  Port=7  Side=Left
  connections:
  Beam xForm/LConn1 -- Column/RConn2
  B/RConn1 -- Base Offset/RConn1
  CUP/RConn1 -- Column Pulleys/LConn1
  Column Pulleys/RConn1 -- Column/RConn1
  Column/LConn1 -- Column Pulleys/RConn2
  CLP/RConn1 -- Column Pulleys/LConn2
  Beam xForm/RConn1 -- Beam/LConn3
  BUP/RConn1 -- Beam Left-End Pulleys/LConn1
  BLP/RConn1 -- Beam Left-End Pulleys/LConn2
  Beam Left-End Pulleys/RConn1 -- Beam/LConn1
  Beam Left-End Pulleys/RConn2 -- Beam/LConn2
  Beam Right-End Pulleys/RConn1 -- BUCP/RConn1
  Beam Right-End Pulleys/LConn1 -- Beam/RConn1
  Beam Right-End Pulleys/LConn2 -- Beam/RConn2
  Beam Right-End Pulleys/LConn3 -- Beam/RConn3
  Beam Right-End Pulleys/RConn2 -- BLCP/RConn1
  Base Offset/LConn1 -- Column/LConn2

== system sm_cable_robot_lib/Frame and Cable Assembly ==
  Frame Assembly : $bdroot/Frame Assembly  frameType=Right-Hand  frameColumnWidth=frameColumnWidth  frameColumnHeight=frameColumnHeight  frameBeamWidth=frameBeamWidth  frameBeamLength=frameBeamLength  bracketWidth=bracketWidth  bracketThickness=bracketThickness  bracketTolerance=bracketTolerance  swivelHoleRadius=swivelHoleRadius  rightAngleBracketWidth=rightBracketWidth  pulleyRadius=pulleyRadius  pulleyThickness=pulleyThickness  pulleyHoleRadius=pulleyHoleRadius  pulleyGrooveDepth=pulleyGrooveDepth  pulleyGrooveWidth=pulleyGrooveWidth  pulleyGrooveAngle=pulleyGrooveAngle  pulleyFrameGap=pulleyFrameGap  frameRho=frameRho  pulleyRho=pulleyRho  pinRho=pinRho  frameColor=frameColor  bracketColor=bracketColor  pulleyColor=pulleyColor  pulleyMarkerColor=pulleyMarkerColor  pinColor=pinColor
  Lower Cable Circuit : Subsystem
      mask Display: image(fullfile(matlabroot,'toolbox','physmod','sm','smdemos','cable_robot','images','sm_cable_robot_lower_cable_circuit.png'));
  Upper Cable Circuit : Subsystem
      mask Display: image(fullfile(matlabroot,'toolbox','physmod','sm','smdemos','cable_robot','images','sm_cable_robot_upper_cable_circuit.png'));
  B : PMIOPort  Side=Left
  UE : PMIOPort  Port=2  Side=Right
  LE : PMIOPort  Port=3  Side=Right
  connections:
  Lower Cable Circuit/LConn1 -- LE/RConn1
  Upper Cable Circuit/RConn1 -- UE/RConn1
  Frame Assembly/RConn1 -- Upper Cable Circuit/LConn1
  Upper Cable Circuit/LConn2 -- Frame Assembly/RConn2
  Upper Cable Circuit/LConn3 -- Frame Assembly/RConn3
  Lower Cable Circuit/RConn4 -- Frame Assembly/LConn4 -- Upper Cable Circuit/LConn4 -- B/RConn1
  Lower Cable Circuit/RConn3 -- Frame Assembly/LConn3
  Lower Cable Circuit/RConn2 -- Frame Assembly/LConn2
  Lower Cable Circuit/RConn1 -- Frame Assembly/LConn1

== system sm_cable_robot_lib/Motor ==
  Flange : sm_lib/Body Elements/Cylindrical Solid  GraphicAmbientColor=[0.15 0.15 0.15 1.0]  BasedOnType=Density  CenterOfMass=[0 0 0]  CenterOfMassUnits=m  GraphicDiffuseColor=flangeColor  CylinderLength=flangeThickness  CylinderLengthUnits=m  CylinderRadius=flangeRadius  CylinderRadiusUnits=m  Density=housingRho  DensityUnits=kg/m^3  DoExposeReferenceFrame=off  GraphicEmissiveColor=[0.0 0.0 0.0 1.0]  ExportEntireGeometry=off  SerializedFrames=<Frames><Frame><Id>Frame1</Id><Value><Name>B</Name><Origin><Source>GeometricFeature</Source><FeatureName>bottom surface</FeatureName></Origin><PrimaryAxis><DefinedDirection>+Z</DefinedDirection><Source>ReferenceFrame</Source><SourceDirection>+Z</SourceDirection><FeatureName></FeatureName></PrimaryAxis><SecondaryAxis><DefinedDirection>+X</DefinedDirection><Source>ReferenceFrame</Source><SourceDirection>+X</SourceDirection><FeatureName></FeatureName></SecondaryAxis></Value></Frame></Frames>  MarkerShape=Sphere  MarkerSize=10  GraphicType=FromGeometry  InertiaType=CalculateFromGeometry  Mass=1  MassUnits=kg  MomentsOfInertia=[1 1 1]  MomentsOfInertiaUnits=kg*m^2  GraphicOpacity=1.0  ProductsOfInertia=[0 0 0]  ProductsOfInertiaUnits=kg*m^2  GraphicShininess=75  GraphicSpecularColor=[0.5 0.5 0.5 1.0]  GraphicVisPropType=SimpleVisualProperties
  Housing : sm_lib/Body Elements/Brick Solid  GraphicAmbientColor=[0.15 0.15 0.15 1.0]  BasedOnType=Density  BrickDimensions=[width height depth]  BrickDimensionUnits=m  CenterOfMass=[0 0 0]  CenterOfMassUnits=m  GraphicDiffuseColor=housingColor  Density=housingRho  DensityUnits=kg/m^3  DoExposeReferenceFrame=off  GraphicEmissiveColor=[0.0 0.0 0.0 1.0]  ExportEntireGeometry=off  SerializedFrames=<Frames><Frame><Id>Frame2</Id><Value><Name>B</Name><Origin><Source>GeometricFeature</Source><FeatureName>-y surface</FeatureName></Origin><PrimaryAxis><DefinedDirection>+Z</DefinedDirection><Source>ReferenceFrame</Source><SourceDirection>+Z</SourceDirection><FeatureName></FeatureName></PrimaryAxis><SecondaryAxis><DefinedDirection>+X</DefinedDirection><Source>ReferenceFrame</Source><SourceDirection>+X</SourceDirection><FeatureName></FeatureName></SecondaryAxis></Value></Frame><Frame><Id>Frame3</Id><Value><Name>F</Name><Origin><Source>GeometricFeature</Source><FeatureName>+z surface</FeatureName></Origin><PrimaryAxis><DefinedDirection>+Z</DefinedDirection><Source>ReferenceFrame</Source><SourceDirection>+Z</SourceDirection><FeatureName></FeatureName></PrimaryAxis><SecondaryAxis><DefinedDirection>+X</DefinedDirection><Source>ReferenceFrame</Source><SourceDirection>+X</SourceDirection><FeatureName></FeatureName></SecondaryAxis></Value></Frame></Frames>  MarkerShape=Sphere  MarkerSize=10  GraphicType=FromGeometry  InertiaType=CalculateFromGeometry  Mass=1  MassUnits=kg  MomentsOfInertia=[1 1 1]  MomentsOfInertiaUnits=kg*m^2  GraphicOpacity=1.0  ProductsOfInertia=[0 0 0]  ProductsOfInertiaUnits=kg*m^2  GraphicShininess=75  GraphicSpecularColor=[0.5 0.5 0.5 1.0]  GraphicVisPropType=SimpleVisualProperties
  Motor Revolute : sm_lib/Joints/Revolute Joint  JointMode=Normal  SenseConstraintForce=off  SenseConstraintForceX=off  SenseConstraintForceY=off  SenseConstraintForceZ=off  SenseConstraintTorque=off  SenseConstraintTorqueX=off  SenseConstraintTorqueY=off  SenseConstraintTorqueZ=off  SenseTotalForce=off  SenseTotalForceX=off  SenseTotalForceY=off  SenseTotalForceZ=off  SenseTotalTorque=off  SenseTotalTorqueX=off  SenseTotalTorqueY=off  SenseTotalTorqueZ=off  CompositeWrenchDir=FollowerOnBase  CompositeWrenchFrame=BaseFrame  EquilibriumPosition=0  EquilibriumPositionUnits=deg  SpringStiffness=0  SpringStiffnessUnits=N*m/deg  DampingCoefficient=0  DampingCoefficientUnits=N*m/(deg/s)  TorqueActuationMode=NoTorque  MotionActuationMode=ComputedMotion  SensePosition=off  SenseVelocity=off  SenseAcceleration=off  SenseTorqueForce=off  SenseLowerLimitTorqueForce=off  SenseUpperLimitTorqueForce=off  LowerLimitSpecify=off  LowerLimitBound=-90  LowerLimitBoundUnits=deg  LowerLimitStiffness=1e4  LowerLimitStiffnessUnits=N*m/deg  LowerLimitDamping=10  LowerLimitDampingUnits=N*m/(deg/s)  LowerLimitTransitionRegionWidth=0.1  LowerLimitTransitionRegionWidthUnits=deg  UpperLimitSpecify=off  UpperLimitBound=90  UpperLimitBoundUnits=deg  UpperLimitStiffness=1e4  UpperLimitStiffnessUnits=N*m/deg  UpperLimitDamping=10  UpperLimitDampingUnits=N*m/(deg/s)  UpperLimitTransitionRegionWidth=0.1  UpperLimitTransitionRegionWidthUnits=deg  PositionTargetSpecify=off  PositionTargetPriority=High  PositionTargetValue=0  PositionTargetValueUnits=deg  VelocityTargetSpecify=off  VelocityTargetPriority=High  VelocityTargetValue=0  VelocityTargetValueUnits=deg/s
  Shaft : sm_lib/Body Elements/Cylindrical Solid  GraphicAmbientColor=[0.15 0.15 0.15 1.0]  BasedOnType=Density  CenterOfMass=[0 0 0]  CenterOfMassUnits=m  GraphicDiffuseColor=shaftColor  CylinderLength=shaftLength  CylinderLengthUnits=m  CylinderRadius=shaftRadius  CylinderRadiusUnits=m  Density=shaftRho  DensityUnits=kg/m^3  DoExposeReferenceFrame=on  GraphicEmissiveColor=[0.0 0.0 0.0 1.0]  ExportEntireGeometry=off  SerializedFrames=<Frames><Frame><Id>Frame1</Id><Value><Name>B</Name><Origin><Source>GeometricFeature</Source><FeatureName>bottom surface</FeatureName></Origin><PrimaryAxis><DefinedDirection>+Z</DefinedDirection><Source>ReferenceFrame</Source><SourceDirection>+Z</SourceDirection><FeatureName></FeatureName></PrimaryAxis><SecondaryAxis><DefinedDirection>+X</DefinedDirection><Source>ReferenceFrame</Source><SourceDirection>+X</SourceDirection><FeatureName></FeatureName></SecondaryAxis></Value></Frame></Frames>  MarkerShape=Sphere  MarkerSize=10  GraphicType=FromGeometry  InertiaType=CalculateFromGeometry  Mass=1  MassUnits=kg  MomentsOfInertia=[1 1 1]  MomentsOfInertiaUnits=kg*m^2  GraphicOpacity=1.0  ProductsOfInertia=[0 0 0]  ProductsOfInertiaUnits=kg*m^2  GraphicShininess=75  GraphicSpecularColor=[0.5 0.5 0.5 1.0]  GraphicVisPropType=SimpleVisualProperties
  B : PMIOPort  Side=Left
  S : PMIOPort  Port=2  Side=Right
  connections:
  Motor Revolute/LConn1 -- Housing/RConn1 -- Flange/LConn1
  Shaft/LConn1 -- Motor Revolute/RConn1
  S/RConn1 -- Shaft/RConn1
  Housing/LConn1 -- B/RConn1

== system sm_cable_robot_lib/Motor Assembly ==
  Motor : $bdroot/Motor  width=motorWidth  height=motorHeight  depth=motorDepth  shaftRadius=motorShaftRadius  shaftLength=motorShaftLength  housingRho=motorHousingRho  shaftRho=motorShaftRho  housingColor=motorHousingColor  flangeColor=motorFlangeColor  shaftColor=motorShaftColor
  Spool : $bdroot/Pulley  radius=spoolRadius  thickness=spoolThickness  holeRadius=motorShaftRadius  grooveDepth=spoolGrooveDepth  grooveWidth=spoolGrooveWidth  grooveAngle=spoolGrooveAngle  rho=spoolRho  color=spoolColor  markerColor=spoolMarkerColor
  Spool Alignment : sm_lib/Frames and Transforms/Rigid Transform  TranslationMethod=None  TranslationStandardOffset=0  TranslationLengthUnit=m  TranslationStandardAxis=+Z  TranslationCartesianOffset=[0 0 0]  TranslationROffset=0  TranslationROffsetUnits=m  TranslationZOffset=0  TranslationZOffsetUnits=m  TranslationThetaOffset=0  TranslationThetaOffsetUnits=deg  RotationMethod=AlignedAxes  RotationAngleUnits=deg  RotationStandardAxis=+Z  RotationAngle=0.0  RotationArbitraryAxis=[0 0 1]  FollAlignAxisA=+Z  BaseAlignAxisA=+Z  FollAlignAxisB=+Y  BaseAlignAxisB=+Y  RotationSequenceAxes=FollowerAxes  RotationSequence=XYX  RotationSequenceAngles=[0 0 0]  RotationSequenceAnglesUnits=deg  RotationMatrix=[1 0 0; 0 1 0; 0 0 1]
  B : PMIOPort  Side=Left
  S : PMIOPort  Port=2  Side=Right
  connections:
  Motor/LConn1 -- B/RConn1
  Spool/LConn1 -- Spool Alignment/LConn1 -- Motor/RConn1
  S/RConn1 -- Spool Alignment/RConn1
